simulink model "sldemo_fuelsys_dd_controller"  (R2021b)
settings: Solver=FixedStepDiscrete  StartTime=0.0  StopTime=10  FixedStep=0.01  RelTol=1e-5  AbsTol=1e-6
values from neighbouring files (symbols this model uses):
  hys = 25.0    [sldemo_fuelsys_dd_controller.sldd]
  max_ego = 1.2    [sldemo_fuelsys_dd_controller.sldd]
  max_press = 0.9375    [sldemo_fuelsys_dd_controller.sldd]
  max_speed = 628.0    [sldemo_fuelsys_dd_controller.sldd]
  max_throt = 88.0    [sldemo_fuelsys_dd_controller.sldd]
  min_press = 0.0625    [sldemo_fuelsys_dd_controller.sldd]
  min_throt = 3.0    [sldemo_fuelsys_dd_controller.sldd]
  PressEst = 0.66451109506242712 0.40057537246380581 0.27077162923530573 0.2046348388305434 0.16218837337748182 0.13507089027241911 0.11253610808285311 0.097096573209803055 0.084644816123708375 0.074166766539525586 0.066404329401423 0.059583991662872149 0.053705753323873048 0.049038488148507725 0.04492523855946047 0.041600795707206269 0.038276352854952053 0.035215332156377753 0.032944577918843157 0.73542424120    [sldemo_fuelsys_dd_controller.sldd]
  PressVect : value not decoded    [sldemo_fuelsys_dd_controller.sldd]
  PumpCon = -0.010768420000000006 0.030750459999999997 0.052019292 0.065700699999999987 0.076070539999999992 0.084118476 0.09144319599999999 0.097613307999999982 0.10327589999999998 0.10860225999999998 0.11345281999999998 0.1181342066666667 0.12264642000000016 0.1269365933333334 0.131123148 0.135161676 0.139200204 0.14318798 0.14702349999999989 0.026704729999999996 0.054584009999999995 0.069445402 0.079429164    [sldemo_fuelsys_dd_controller.sldd]
  RampRateKiX : value not decoded    [sldemo_fuelsys_dd_controller.sldd]
  RampRateKiY : value not decoded    [sldemo_fuelsys_dd_controller.sldd]
  RampRateKiZ : value not decoded    [sldemo_fuelsys_dd_controller.sldd]
  SpeedEst = 423.780479257259 471.77707643652047 564.94153173664483 703.27384515763185 889.115473646033 1085.6871282532522 1292.9888089792896 1509.224946867465 1726.8856607331168 1945.9709505762448 2164.71831215501 2382.3898758165424 2598.9856415608424 2812.3140461970188 3023.6400813709542 3232.9637470826474 3436.1353600597686 3639.3069730368893 3835.4161363935882 4024.4628501298644 4213.5095638661405 4402.556    [sldemo_fuelsys_dd_controller.sldd]
  SpeedVect : value not decoded    [sldemo_fuelsys_dd_controller.sldd]
  st_range = 0.0001    [sldemo_fuelsys_dd_controller.sldd]
  ThrotEst = 0.0 0.0 0.0 0.0 0.0 0.0 0.059371351459993185 0.37601855924662353 0.64679219391594289 0.88560631059796346 1.0578898155263028 1.217140421226361 1.3633581276981388 2.3428818771619091 3.2073236691363545 3.7873726382961488 4.3674216074559418 4.9091415297603671 5.3358743114986886 0.0 0.0 0.0 0.0 0.0 0.0 0.20779973010997618 1.3160649573631824 2.2637726787058003 3.0996220870928726 3.7026143543420598 4.259    [sldemo_fuelsys_dd_controller.sldd]
  ThrotVect : value not decoded    [sldemo_fuelsys_dd_controller.sldd]
  zero_thresh = 250.0    [sldemo_fuelsys_dd_controller.sldd]
undefined symbols (not defined in the file or in its folder): DiscIntNeverNeededParam, sld_FuelModes, sldvsubsys
libraries: simulink x2
settings Model: DataDictionary=sldemo_fuelsys_dd_controller.sldd  EnableAccessToBaseWorkspace=off  Creator=The MathWorks, Inc.  LastModifiedBy=zmahi
settings SolverCC: AutoScaleAbsTol=off  AlgebraicLoopSolver=TrustRegion
settings DataIOCC: SaveFormat=StructureWithTime  SaveOutput=off  SaveTime=off  ReturnWorkspaceOutputs=off  SignalLoggingName=sldemo_fuelsys_output
settings OptimizationCC: DefaultParameterBehavior=Inlined  UseDivisionForNetSlopeComputation=UseDivisionForReciprocalsOfIntegersOnly  InlineInvariantSignals=on  EnhancedBackFolding=on  StrengthReduction=on  PassReuseOutputArgsThreshold=0  ExpressionDepthLimit=2147483647  StateBitsets=on  DataBitsets=on  EfficientFloat2IntCast=on
settings DebuggingCC: SignalInfNanChecking=error  SaveWithParameterizedLinksMsg=none  UnderspecifiedInitializationDetection=Classic  CheckExecutionContextPreStartOutputMsg=on  IntegerOverflowMsg=none  ParameterDowncastMsg=warning  ParameterOverflowMsg=none  ParameterPrecisionLossMsg=none  UnderSpecifiedDataTypeMsg=warning  FcnCallInpInsideContextMsg=warning  UniqueDataStoreMsg=error  BusObjectLabelMismatch=error  StateNameClashWarn=warning  StrictBusMsg=ErrorOnBusTreatedAsVector  SFUnexpectedBacktrackingDiag=warning  SFNoUnconditionalDefaultTransitionDiag=warning  SFExecutionAtInitializationDiag=none  SFMachineParentedDataDiag=warning  IntegerSaturationMsg=none  ArithmeticOperatorsInVariantConditions=warning
settings ModelReferenceCC: ModelReferenceNumInstancesAllowed=Single  PropagateSignalLabelsOutOfModel=off
settings SFSimCC: SimUseLocalCustomCode=off  SimParseCustomCode=off  MATLABDynamicMemAlloc=off  CustomCodeUndefinedFunction=UseInterfaceOnly
settings RTWCC: GenCodeOnly=on  GenerateReport=on  RTWVerbose=off  RTWUseLocalCustomCode=off  LaunchReport=on
settings CodeAppCC: ForceParamTrailComments=on  StateflowObjectComments=on
settings GRTTargetCC: TargetLangStandard=C89/C90 (ANSI)
settings ConfigComp: CovScope=Subsystem  CovPath=control_logic  CovMetricSettings=dw  CovSaveCumulativeToWorkspaceVar=on  CovSaveSingleToWorkspaceVar=on  CovExternalEMLEnable=off  CovSFcnEnable=off

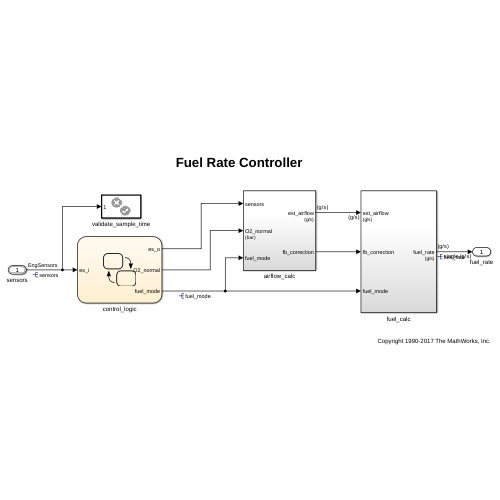
[thumbnail: Simulink's stored preview of the top-level diagram]
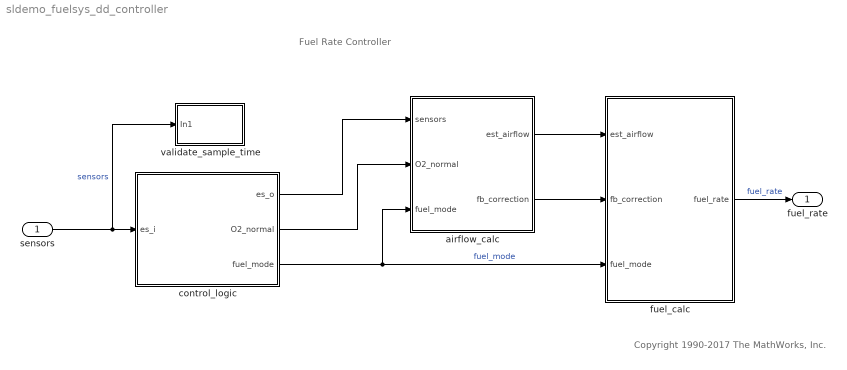
== system sldemo_fuelsys_dd_controller ==
  note: Copyright 1990-2017 The MathWorks, Inc.
  note: Fuel Rate Controller
  sensors : Inport  OutDataTypeStr=Bus: EngSensors  PortDimensions=1  SampleTime=[0.01,0]  BusOutputAsStruct=on
  airflow_calc : Subsystem
  control_logic : Stateflow chart  Description=Stateflow diagram to determine control system operating mode  TreatAsAtomicUnit=on
  fuel_calc : Subsystem
  validate_sample_time : Subsystem  Tag=VerificationSubsystem  DisableCoverage=on  LoadFcn=sldvsubsys('check')  TreatAsAtomicUnit=on  SimViewingDevice=on  mask(VerificationSubsystem){}
      mask init:
      | sldvsubsys('maskInit');
      settings: CopyFcn=sldvsubsys('copy');  OpenFcn=open_system(gcb,'force');
      settings: PreSaveFcn=|
      | set_param(gcb,'SimViewingDevice','on');
      | sldvsubsys('check');
      mask Help: helpview(fullfile(docroot,'toolbox','sldv','sldv.map'),'verificationsubsystem')
      mask Display: image(imread('sldvicon_versubsys.png','BackGroundColor',[1 1 1]),'center');
  fuel_rate : Outport  OutDataTypeStr=s16En7  Unit=g/s  PortDimensions=1  SampleTime=[0.01,0]  VectorParamsAs1DForOutWhenUnconnected=off
  wires:
  fuel_calc/1(fuel_rate) -> fuel_rate/1  "fuel_rate"
  airflow_calc/1(est_airflow) -> fuel_calc/1(est_airflow)
  sensors/1 -> validate_sample_time/1(In1), control_logic/1(es_i)  "sensors"
  control_logic/3(fuel_mode) -> fuel_calc/3(fuel_mode), airflow_calc/3(fuel_mode)  "fuel_mode"
  control_logic/1(es_o) -> airflow_calc/1(sensors)
  control_logic/2(" O2_normal") -> airflow_calc/2(O2_normal)
  airflow_calc/2(fb_correction) -> fuel_calc/2(fb_correction)

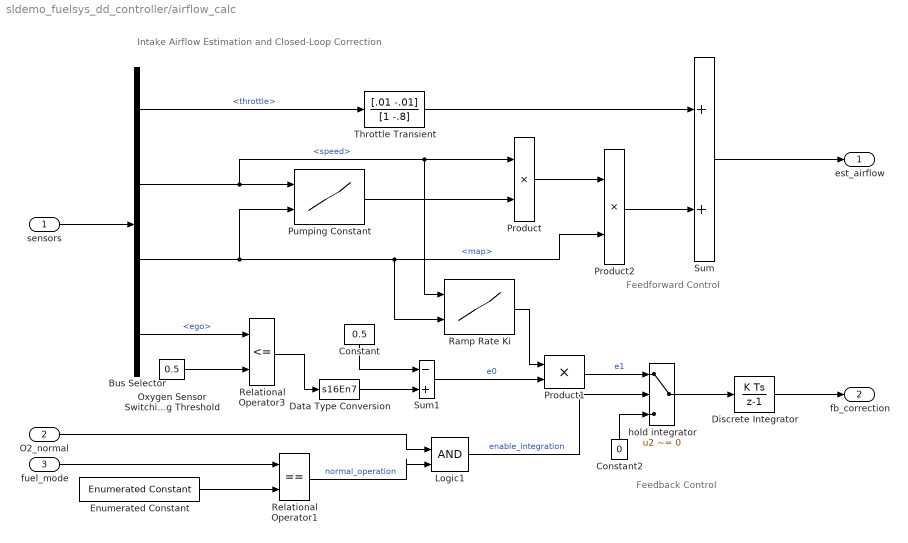
== system sldemo_fuelsys_dd_controller/airflow_calc ==
  note: Feedforward Control
  note: Feedback Control
  note: Intake Airflow Estimation and Closed-Loop Correction
  sensors : Inport
  O2_normal : Inport  Port=2
  fuel_mode : Inport  Port=3
  Bus Selector : BusSelector  OutputSignals=throttle,speed,map,ego
  Constant : Constant  Value=0.5  OutDataTypeStr=s16En7
  Constant2 : Constant  Value=0  OutDataTypeStr=uint8
  Data Type Conversion : DataTypeConversion  OutDataTypeStr=s16En7  RndMeth=Simplest
  Discrete Integrator : DiscreteIntegrator  SampleTime=-1  OutDataTypeStr=s16En15  RndMeth=Simplest  ICPrevOutput=DiscIntNeverNeededParam  ICPrevScaledInput=DiscIntNeverNeededParam
  Enumerated Constant : simulink/Sources/Enumerated Constant  OutDataTypeStr=Enum: sld_FuelModes  Value=sld_FuelModes.LOW  SampleTime=.01
  Logic1 : Logic  IconShape=distinctive  AllPortsSameDT=off  OutDataTypeStr=boolean
  Oxygen Sensor Switching Threshold : Constant  Value=0.5  OutDataTypeStr=s16En7
  Product : Product  OutDataTypeStr=s16En7  RndMeth=Simplest
  Product1 : Product  OutDataTypeStr=s16En15  RndMeth=Simplest
  Product2 : Product  OutDataTypeStr=s16En7  RndMeth=Simplest
  Pumping Constant : Lookup_n-D  BreakpointsForDimension1=SpeedVect  BreakpointsForDimension2=PressVect  IndexSearchMethod=Linear search  Table=PumpCon  ExtrapMethod=Clip  UseLastTableValue=on  OutDataTypeStr=s16En15  RndMeth=Simplest
      settings: InputPortMap=u0,u1
  Ramp Rate Ki : Lookup_n-D  BreakpointsForDimension1=RampRateKiX  BreakpointsForDimension2=RampRateKiY  IndexSearchMethod=Linear search  Table=RampRateKiZ  ExtrapMethod=Clip  UseLastTableValue=on  OutDataTypeStr=s16En15  RndMeth=Simplest
      settings: InputPortMap=u0,u1
  Relational Operator1 : RelationalOperator  Operator===  OutDataTypeStr=boolean  RndMeth=Nearest  InputSameDT=on
  Relational Operator3 : RelationalOperator  Operator=<=  OutDataTypeStr=boolean  RndMeth=Nearest
  Sum : Sum  Inputs=2  OutDataTypeStr=s16En7  RndMeth=Simplest
  Sum1 : Sum  Inputs=-+  OutDataTypeStr=s16En15  RndMeth=Simplest
  Throttle Transient : DiscreteFilter  Numerator=[.01 -.01]  Denominator=[1 -.8]  a0EqualsOne=on  OutDataTypeStr=s16En7  RndMeth=Simplest
  hold integrator : Switch  Criteria=u2 ~= 0  Threshold=1  OutDataTypeStr=s16En15  RndMeth=Simplest
  est_airflow : Outport  Unit=g/s  VectorParamsAs1DForOutWhenUnconnected=off
  fb_correction : Outport  Port=2  VectorParamsAs1DForOutWhenUnconnected=off
  wires:
  fuel_mode/1 -> Relational Operator1/1
  Enumerated Constant/1 -> Relational Operator1/2
  O2_normal/1 -> Logic1/1
  Product2/1 -> Sum/2
  Product/1 -> Product2/1
  Bus Selector/4 -> Relational Operator3/1  "<ego>"
  Bus Selector/3 -> Pumping Constant/2, Ramp Rate Ki/2, Product2/2  "<map>"
  Data Type Conversion/1 -> Sum1/2
  Relational Operator3/1 -> Data Type Conversion/1
  Sum1/1 -> Product1/2  "e0"
  Logic1/1 -> hold integrator/2  "enable_integration"
  hold integrator/1 -> Discrete Integrator/1
  Product1/1 -> hold integrator/1  "e1"
  Constant2/1 -> hold integrator/3
  Ramp Rate Ki/1 -> Product1/1
  Constant/1 -> Sum1/1
  Oxygen Sensor Switching Threshold/1 -> Relational Operator3/2
  Relational Operator1/1 -> Logic1/2  "normal_operation"
  Bus Selector/1 -> Throttle Transient/1  "<throttle>"
  Sum/1 -> est_airflow/1
  Throttle Transient/1 -> Sum/1
  Bus Selector/2 -> Pumping Constant/1, Ramp Rate Ki/1, Product/1  "<speed>"
  Pumping Constant/1 -> Product/2
  sensors/1 -> Bus Selector/1
  Discrete Integrator/1 -> fb_correction/1

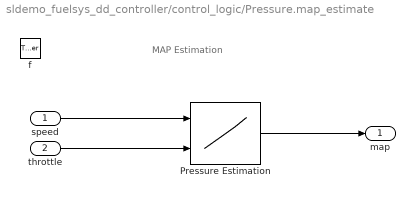
== system sldemo_fuelsys_dd_controller/control_logic/Pressure.map_estimate ==
  note: MAP Estimation
  speed : Inport  OutDataTypeStr=s16En3
  throttle : Inport  Port=2  OutDataTypeStr=s16En3
  f : TriggerPort  TriggerType=function-call  VariantControl=(inherit)
      settings: CopyFcn=Stateflow.SLINSF.SimulinkMan.removeBlockPreDeleteFcn  PreDeleteFcn=Stateflow.SLINSF.SimulinkMan.unsafePredeleteFcn
  Pressure Estimation : Lookup_n-D  BreakpointsForDimension1=SpeedVect  BreakpointsForDimension2=ThrotVect  IndexSearchMethod=Linear search  Table=PressEst  ExtrapMethod=Clip  UseLastTableValue=on  OutDataTypeStr=u8En7  RndMeth=Simplest
      settings: InputPortMap=u0,u1
  map : Outport  VectorParamsAs1DForOutWhenUnconnected=off
  wires:
  Pressure Estimation/1 -> map/1
  throttle/1 -> Pressure Estimation/2
  speed/1 -> Pressure Estimation/1

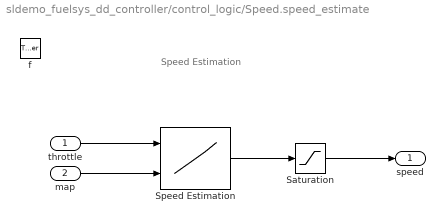
== system sldemo_fuelsys_dd_controller/control_logic/Speed.speed_estimate ==
  note: Speed Estimation
  throttle : Inport  OutDataTypeStr=s16En3
  map : Inport  Port=2  OutDataTypeStr=u8En7
  f : TriggerPort  TriggerType=function-call  VariantControl=(inherit)
      settings: CopyFcn=Stateflow.SLINSF.SimulinkMan.removeBlockPreDeleteFcn  PreDeleteFcn=Stateflow.SLINSF.SimulinkMan.unsafePredeleteFcn
  Saturation : Saturate  UpperLimit=max_speed  LowerLimit=0  OutDataTypeStr=s16En3
  Speed Estimation : Lookup_n-D  BreakpointsForDimension1=ThrotVect  BreakpointsForDimension2=PressVect  IndexSearchMethod=Linear search  Table=SpeedEst  ExtrapMethod=Clip  UseLastTableValue=on  OutDataTypeStr=s16En3  RndMeth=Simplest
      settings: InputPortMap=u0,u1
  speed : Outport  VectorParamsAs1DForOutWhenUnconnected=off
  wires:
  Saturation/1 -> speed/1
  map/1 -> Speed Estimation/2
  throttle/1 -> Speed Estimation/1
  Speed Estimation/1 -> Saturation/1

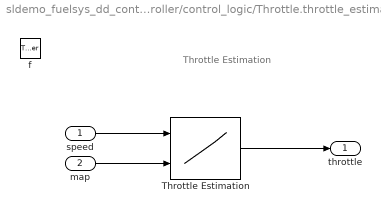
== system sldemo_fuelsys_dd_controller/control_logic/Throttle.throttle_estimate ==
  note: Throttle Estimation
  speed : Inport  OutDataTypeStr=s16En3
  map : Inport  Port=2  OutDataTypeStr=u8En7
  f : TriggerPort  TriggerType=function-call  VariantControl=(inherit)
      settings: CopyFcn=Stateflow.SLINSF.SimulinkMan.removeBlockPreDeleteFcn  PreDeleteFcn=Stateflow.SLINSF.SimulinkMan.unsafePredeleteFcn
  Throttle Estimation : Lookup_n-D  BreakpointsForDimension1=SpeedVect  BreakpointsForDimension2=PressVect  IndexSearchMethod=Linear search  Table=ThrotEst  ExtrapMethod=Clip  UseLastTableValue=on  OutDataTypeStr=s16En7  RndMeth=Simplest
      settings: InputPortMap=u0,u1
  throttle : Outport  VectorParamsAs1DForOutWhenUnconnected=off
  wires:
  Throttle Estimation/1 -> throttle/1
  map/1 -> Throttle Estimation/2
  speed/1 -> Throttle Estimation/1

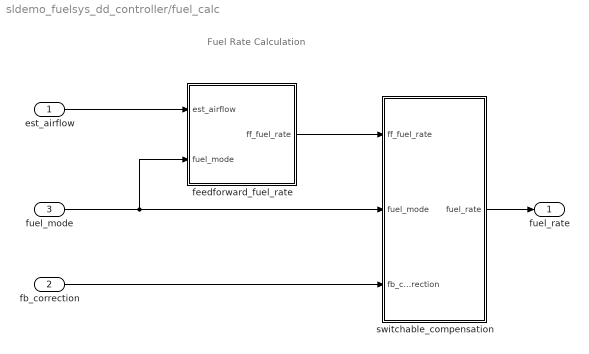
== system sldemo_fuelsys_dd_controller/fuel_calc ==
  note: Fuel Rate Calculation
  est_airflow : Inport  Unit=g/s
  fb_correction : Inport  Port=2
  fuel_mode : Inport  Port=3
  feedforward_fuel_rate : Subsystem
  switchable_compensation : Subsystem
  fuel_rate : Outport  Unit=g/s  VectorParamsAs1DForOutWhenUnconnected=off
  wires:
  feedforward_fuel_rate/1(ff_fuel_rate) -> switchable_compensation/1(ff_fuel_rate)
  fb_correction/1 -> switchable_compensation/3(fb_correction)
  switchable_compensation/1(fuel_rate) -> fuel_rate/1
  fuel_mode/1 -> switchable_compensation/2(fuel_mode), feedforward_fuel_rate/2(fuel_mode)
  est_airflow/1 -> feedforward_fuel_rate/1(est_airflow)

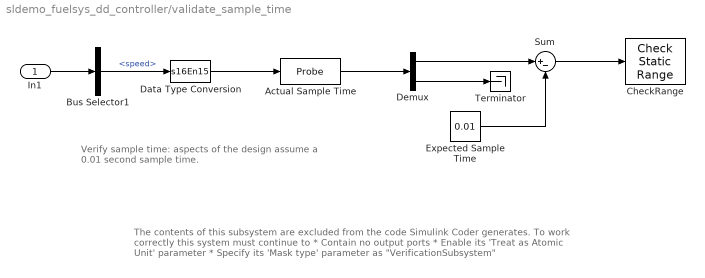
== system sldemo_fuelsys_dd_controller/validate_sample_time ==
  note: Verify sample time: aspects of the design
      | assume a 0.01 second sample time.
  note: The contents of this subsystem are excluded from the code Simulink Coder generates.
      |
      | To work correctly this system must continue to
      | * Contain no output ports
      | * Enable its 'Treat as Atomic Unit' parameter
      | * Specify its 'Mask type' parameter as "VerificationSubsystem"
  In1 : Inport
  Actual Sample Time : Probe  ProbeWidth=off  ProbeComplexSignal=off  ProbeSampleTimeDataType=Same as input
  Bus Selector1 : BusSelector  OutputSignals=speed
  CheckRange : simulink/Model Verification/Check  Static Range  Description=-st_range < u < st_range  max=st_range  max_included=off  min=-st_range  min_included=off  enabled=on  stopWhenAssertionFail=on  export=off  icon=graphic
      settings: SourceProductBaseCode=SL
  Data Type Conversion : DataTypeConversion  OutDataTypeStr=s16En15
  Demux : Demux  Outputs=2
  Expected Sample Time : Constant  Value=0.01  OutDataTypeStr=s16En15
  Sum : Sum  Inputs=|+-  OutDataTypeStr=Inherit: Same as first input
  Terminator : Terminator
  wires:
  Data Type Conversion/1 -> Actual Sample Time/1
  Sum/1 -> CheckRange/1
  Expected Sample Time/1 -> Sum/2
  Demux/1 -> Sum/1
  Demux/2 -> Terminator/1
  Bus Selector1/1 -> Data Type Conversion/1  "<speed>"
  Actual Sample Time/1 -> Demux/1
  In1/1 -> Bus Selector1/1

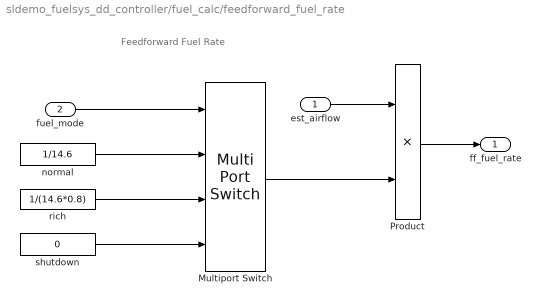
== system sldemo_fuelsys_dd_controller/fuel_calc/feedforward_fuel_rate ==
  note: Feedforward Fuel Rate
  est_airflow : Inport
  fuel_mode : Inport  Port=2
  Multiport Switch : MultiPortSwitch  DataPortOrder=Specify indices  DataPortIndices={sld_FuelModes.LOW, sld_FuelModes.RICH, sld_FuelModes.DISABLED}  OutDataTypeStr=s16En7  RndMeth=Simplest
  Product : Product  OutDataTypeStr=s16En7  RndMeth=Simplest
  normal : Constant  Value=1/14.6  OutDataTypeStr=s16En7
  rich : Constant  Value=1/(14.6*0.8)  OutDataTypeStr=s16En7
  shutdown : Constant  Value=0  OutDataTypeStr=s16En7
  ff_fuel_rate : Outport  VectorParamsAs1DForOutWhenUnconnected=off
  wires:
  shutdown/1 -> Multiport Switch/4
  normal/1 -> Multiport Switch/2
  Multiport Switch/1 -> Product/2
  Product/1 -> ff_fuel_rate/1
  est_airflow/1 -> Product/1
  fuel_mode/1 -> Multiport Switch/1
  rich/1 -> Multiport Switch/3

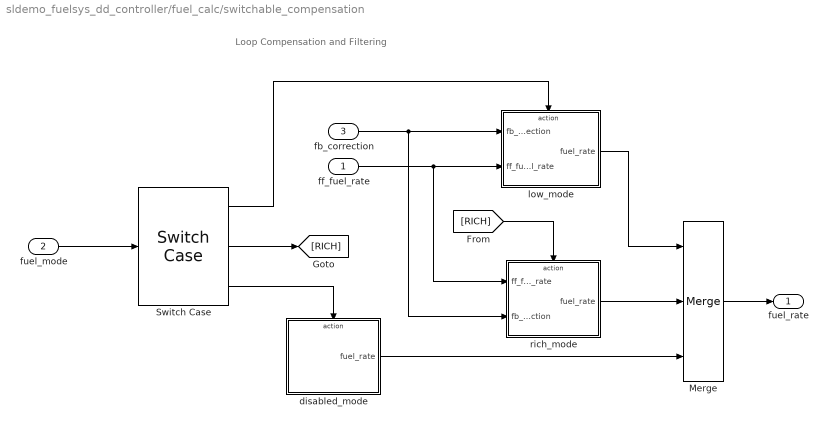
== system sldemo_fuelsys_dd_controller/fuel_calc/switchable_compensation ==
  note: Loop Compensation and Filtering
  ff_fuel_rate : Inport
  fuel_mode : Inport  Port=2
  fb_correction : Inport  Port=3
  Merge : Merge  Inputs=3
  Switch Case : SwitchCase  CaseConditions={sld_FuelModes.LOW, sld_FuelModes.RICH}
  disabled_mode : Subsystem  TreatAsAtomicUnit=on
  low_mode : Subsystem  TreatAsAtomicUnit=on
  rich_mode : Subsystem  TreatAsAtomicUnit=on
  fuel_rate : Outport  VectorParamsAs1DForOutWhenUnconnected=off
  wires:
  Merge/1 -> fuel_rate/1
  low_mode/1(fuel_rate) -> Merge/1
  disabled_mode/1(fuel_rate) -> Merge/3
  rich_mode/1(fuel_rate) -> Merge/2
  Switch Case/3 -> disabled_mode/Action
  [RICH] -> rich_mode/Action
  Switch Case/2 -> [RICH]
  Switch Case/1 -> low_mode/Action
  fb_correction/1 -> low_mode/1(fb_correction), rich_mode/2(fb_correction)
  ff_fuel_rate/1 -> low_mode/2(ff_fuel_rate), rich_mode/1(ff_fuel_rate)
  fuel_mode/1 -> Switch Case/1

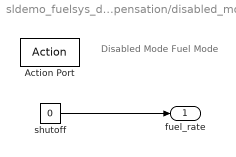
== system sldemo_fuelsys_dd_controller/fuel_calc/switchable_compensation/disabled_mode ==
  note: Disabled Mode Fuel Mode
  Action Port : ActionPort  ActionPortLabel=default:
  shutoff : Constant  Value=0  OutDataTypeStr=Inherit: Inherit via back propagation
  fuel_rate : Outport  InitialOutput=0  VectorParamsAs1DForOutWhenUnconnected=off
  wires:
  shutoff/1 -> fuel_rate/1

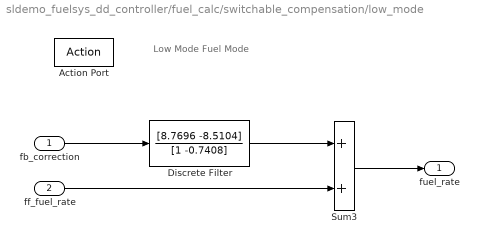
== system sldemo_fuelsys_dd_controller/fuel_calc/switchable_compensation/low_mode ==
  note: Low Mode Fuel Mode
  fb_correction : Inport
  ff_fuel_rate : Inport  Port=2
  Action Port : ActionPort  ActionPortLabel=case [ LOW ]:
  Discrete Filter : DiscreteFilter  Numerator=[8.7696 -8.5104]  Denominator=[1 -0.7408]  a0EqualsOne=on  RndMeth=Simplest  OutDataTypeStr=Inherit: Same as input
  Sum3 : Sum  OutDataTypeStr=s16En7  RndMeth=Simplest
  fuel_rate : Outport  InitialOutput=0  VectorParamsAs1DForOutWhenUnconnected=off
  wires:
  fb_correction/1 -> Discrete Filter/1
  Sum3/1 -> fuel_rate/1
  Discrete Filter/1 -> Sum3/1
  ff_fuel_rate/1 -> Sum3/2

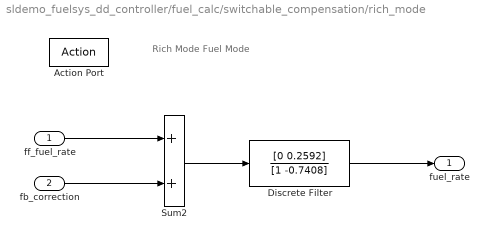
== system sldemo_fuelsys_dd_controller/fuel_calc/switchable_compensation/rich_mode ==
  note: Rich Mode Fuel Mode
  ff_fuel_rate : Inport
  fb_correction : Inport  Port=2
  Action Port : ActionPort  ActionPortLabel=case [ RICH ]:
  Discrete Filter : DiscreteFilter  Numerator=[0 0.2592]  Denominator=[1 -0.7408]  a0EqualsOne=on  RndMeth=Simplest  OutDataTypeStr=Inherit: Same as input
  Sum2 : Sum  OutDataTypeStr=s16En7  RndMeth=Simplest
  fuel_rate : Outport  InitialOutput=0  VectorParamsAs1DForOutWhenUnconnected=off
  wires:
  Discrete Filter/1 -> fuel_rate/1
  Sum2/1 -> Discrete Filter/1
  ff_fuel_rate/1 -> Sum2/1
  fb_correction/1 -> Sum2/2

== stateflow chart sldemo_fuelsys_dd_controller/control_logic ==
  state O2 [parallel]
    settings: executionOrder=1  description=This state determines the validity of the exhaust gas oxygen sensor (EGO) data.
    state A
      du:
      es_o.ego = es_i.ego;
      state O2_warmup
        settings: description=The EGO sensor must come up to temperature before its data is reliable.
      state O2_normal
        settings: description=Normal EGO sensor operation gives a reliable indication of excess oxygen in the exhaust gas, from which air/fuel mixture can be inferred.
      state O2_failure
        settings: description=The EGO sensor has failed.
      (default) -> O2_warmup
      O2_warmup -> O2_normal : [after(480,tick)]
        settings: description=The value for sufficient warm up to operational temperature (nominally 4.8 seconds).
      O2_failure -> O2_normal : [es_i.ego < max_ego] / Fail.DEC;
      O2_normal -> O2_failure : [es_i.ego > max_ego] / Fail.INC;
        settings: description=The failure condition is indicated by excessive output voltage.
    (default) -> A
  state Pressure [parallel]
    settings: executionOrder=2  description=This state assesses the validity of the manifold absolute pressure (MAP) sensor.
    state normal
      du:
      es_o.map = es_i.map;
      settings: description=The manifold pressure sensor gives a reliable indication of absolute pressure (MAP).
    state fail
      du:
      es_o.map = map_estimate(es_i.speed, es_i.throttle);
      settings: description=The pressure sensor (manifold, or MAP) no longer produces reliable data.
    state map = map_estimate(speed, throttle) [function]
    (default) -> Pressure.normal
    Pressure.fail -> Pressure.normal : [es_i.map > min_press & ...
        | es_i.map < max_press] /
        | Fail.DEC;
    Pressure.normal -> Pressure.fail : [es_i.map > max_press | ...
        | es_i.map < min_press] /
        | Fail.INC;
  state Throttle [parallel]
    settings: executionOrder=3  description=This state determines the validity of the throttle sensor signal.
    state normal
      du:
      es_o.throttle = es_i.throttle;
      settings: description=The throttle sensor gives a reliable indication of the angle of the throttle plate.
    state fail
      du:
      es_o.throttle = throttle_estimate(es_i.speed,es_i.map);
      settings: description=Signal levels indicate that the throttle sensor data is no longer valid.
    state throttle = throttle_estimate(speed, map) [function]
    (default) -> Throttle.normal
    Throttle.fail -> Throttle.normal : [es_i.throttle >  min_throt & ...
        | es_i.throttle < max_throt] /
        | Fail.DEC;
    Throttle.normal -> Throttle.fail : [es_i.throttle> max_throt | ...
        | es_i.throttle < min_throt] /
        | Fail.INC;
      settings: description=A failure is indicated by data which is outside the expected range, typically due to an open or short circuit.
  state Speed [parallel]
    settings: executionOrder=4  description="This state infers the validity of the speed sensor data.  A failure is indicated by the presence of manifold vacuum at zero speed."
    state normal
      du:
      es_o.speed = es_i.speed;
      settings: description=The speed sensor data accurately represents the engine speed.
    state fail
      du:
      es_o.speed = speed_estimate(es_i.throttle, es_i.map);
      settings: description=The engine speed data is no longer available.
    state speed = speed_estimate(throttle, map) [function]
    (default) -> Speed.normal
    Speed.fail -> Speed.normal : [es_i.speed > 0C] /
        | Fail.DEC;
    Speed.normal -> Speed.fail : [es_i.speed == 0C & ...
        | es_i.map < zero_thresh] /
        | Fail.INC;
      settings: description="Loss of a reliable speed sensor signal will indicate zero speed.  This is deemed invalid when the manifold vacuum indicates otherwise."
  state Fail [parallel]
    settings: executionOrder=5  description=This state maintains a count of the number of sensors in failure mode.
    state Multi
      settings: description=This state represents any of the conditions in which more than one sensor is in failure mode.
      state Three
        settings: description=Three of the engine sensors have failed.
      state Four
        settings: description=All four of the engine sensors have failed.
      state Two
        settings: description=Two of the engine sensors have failed.
      Three -> Four [order 1] : INC
      Two -> Three [order 2] : INC
      Four -> Three : DEC
      Three -> Two [order 2] : DEC
    state One
      settings: description=One of the engine sensors has failed.
    state None
      settings: description=Zero failures; all sensors are operational.
    (default) -> None
    None -> One : INC
    One -> Two [order 1] : INC
    Two -> One [order 1] : DEC
    One -> None [order 2] : DEC
  state Fueling_Mode [parallel]
    settings: executionOrder=6  description=This state interprets the other states in the chart to directly control the fueling mode.
    state Fuel_Disabled
      en:
      fuel_mode = DISABLED;
      settings: description=The fuel is completely shut off while in this state.
      state Overspeed
        settings: description=The speed is dangerously high, so shut off the fuel.
      state Shutdown
        settings: description=Cut off system operation due to multiple sensor failures.
      Overspeed -> (junction 67) : [in(Speed.normal) & ...
          | es_i.speed < (max_speed - hys)]
      (junction 67) -> Shutdown [order 2] : [in(Fail.Multi)]
    state Running
      settings: description=The fuel is actively controlled while in this state.
      (history)
      state Low_Emissions
        en:
        fuel_mode = LOW;
        (history)
        state Warmup
          settings: description="The sensors are all operational, but the oxygen (EGO) sensor is warming up.  We'll target a stoichiometric ratio, nonetheless, but won't close the loop around exhaust gas oxygen."
        state Normal
          settings: description=All sensors are in correct operating modes, so effective closed-loop mixture control can be used.
        Warmup -> (junction 68) : [in(O2.A.O2_normal)]
        (junction 68) -> Normal [order 2]
      state Rich_Mixture
        en:
        fuel_mode = RICH;
        settings: description=This mode enriches the mixture, lowering the air/fuel ratio.
        state Single_Failure
          settings: description=Continue uninterrupted engine operation, but with a richer mixture.
      (junction 68) -> Single_Failure [order 1] : [in(Fail.One)]
      Normal -> Single_Failure : [in(Fail.One)]
      Single_Failure -> Normal : [in(Fail.None)]
    (default) -> Warmup : {es_o = es_i;}
      settings: description=Need to copy the sensors to the output on entry since the individual elements of the bus signal are only updated in the during function.
    Running -> Overspeed [order 2] : [es_i.speed > max_speed]
    (junction 67) -> Running [order 1] : [!in(Fail.Multi)]
    Running -> Shutdown [order 1] : enter(Fail.Multi)
    Shutdown -> Rich_Mixture : exit(Fail.Multi)
  data: speed function_input s16En3; throttle function_input s16En3; map function_output; speed function_input s16En3; map function_input u8En7; throttle function_output; throttle function_input s16En3; map function_input u8En7; speed function_output; es_o output EngSensors; O2_normal output boolean; max_ego parameter s16En7 [0..2]; max_press parameter u8En7 [0..2]; min_press parameter u8En7 [0..2]; min_throt parameter s16En3 [0..120]; max_throt parameter s16En3 [0..120]; zero_thresh parameter u8En7 [0..450]; max_speed parameter s16En3 [0..1000]; hys parameter s16En3 [0..1000]; es_i input EngSensors; fuel_mode output Enum: sld_FuelModes [1..3] =sld_FuelModes.LOW
  data es_o settings: description=Bus containing the sensor data.
  data max_ego settings: description=Parameter represents the upper end of the EGO sensor range.
  data max_press settings: description=Parameter represents the upper limt of valid pressure readings.
  data min_press settings: description=Parameter for the lower end of the valid pressure sensor range.
  data min_throt settings: description=Minimum valid throttle angle.
  data max_throt settings: description=Parameter to indicate the maximum valid throttle angle reading.
  data zero_thresh settings: description=Minimum manifold pressure expected at zero speed.
  data max_speed settings: description=Parameter for the upper end of the safe engine speed range.
  data hys settings: description=Hysteresis in the upper speed limit to avoid chatter at the threshold.
  data es_i settings: description=Bus containing the sensor data.
  data fuel_mode settings: description=Fuel control mode: LOW = stoichiometric mixture, RICH = rich mixture, DISABLED = shut down
  events: DEC local EITHER_EDGE_EVENT; INC local EITHER_EDGE_EVENT
